simulink model "Frame"  (R2021b)
settings: Solver=FixedStepAuto  StartTime=0.0  StopTime=10  FixedStep=Ts  RelTol=1e-3
model workspace (MAT data in the model file):
  Ts = 0.005
values from neighbouring files (symbols this model uses):
  CODE = str2num(app.InsrerlecodebarresvirguleEditField.Value)    [cao.m]
undefined symbols (not defined in the file or in its folder): alpha_c, amp, AnimActive, couple, courbure, dx_c, dz_c, F_s, filtre, freq, I_0, J_s, photod, ref, theta_c, w_0
libraries: simulink x2
settings Model: Creator=GUBED49  LastModifiedBy=billy
settings DataIOCC: SaveFormat=Array  SignalLogging=off  DSMLogging=off  ReturnWorkspaceOutputs=off

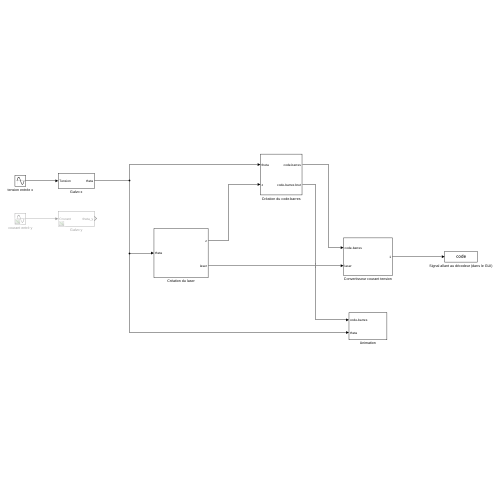
[thumbnail: Simulink's stored preview of the top-level diagram]
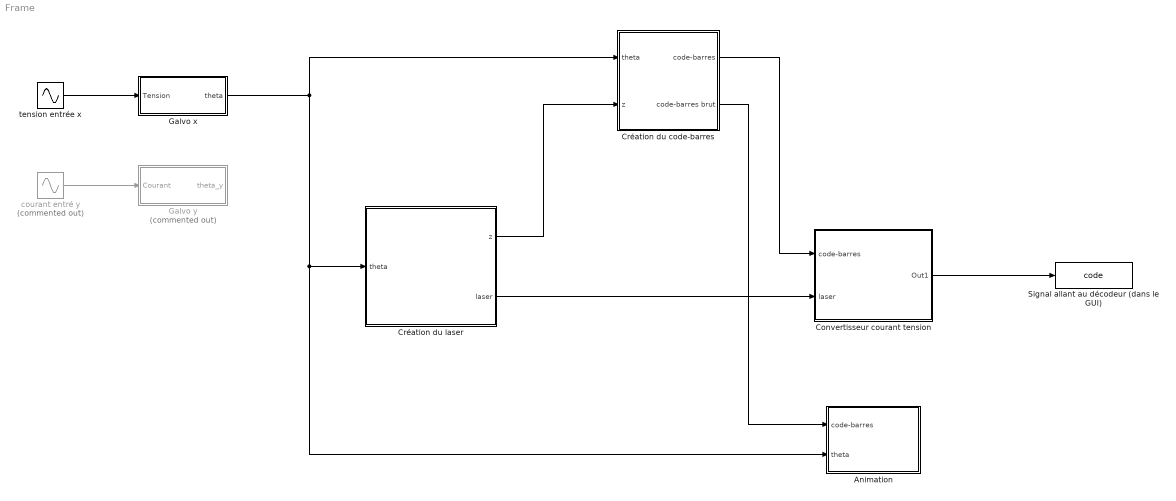
== system Frame ==
  Animation : Subsystem
  Convertisseur courant tension : Subsystem
  Création du code-barres : Subsystem
  Création du laser : Subsystem
  Galvo x : Subsystem
  Galvo y : Subsystem  Commented=on
  Signal allant au décodeur (dans le GUI) : ToWorkspace  VariableName=code  SampleTime=-1
  courant entré y : Sin  Commented=on  Amplitude=amp  Frequency=freq*2*pi  SampleTime=0
  tension entrée x : Sin  Amplitude=amp  Frequency=freq  SampleTime=0
  wires:
  tension entrée x/1 -> Galvo x/1(Tension)
  Galvo x/1(theta) -> Animation/2(theta), Création du laser/1(theta), Création du code-barres/1(theta)
  Création du laser/1(z) -> Création du code-barres/2(z)
  Création du code-barres/1(code-barres) -> Convertisseur courant tension/1(code-barres)
  Création du laser/2(laser) -> Convertisseur courant tension/2(laser)
  Convertisseur courant tension/1(Out1) -> Signal allant au décodeur (dans le GUI)/1
  courant entré y/1 -> Galvo y/1(Courant)
  Création du code-barres/2(code-barres brut) -> Animation/1(code-barres)

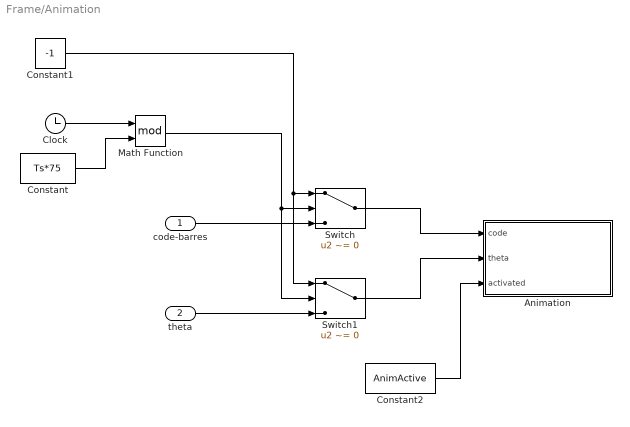
== system Frame/Animation ==
  code-barres : Inport
  theta : Inport  Port=2
  Animation : MATLAB Function  TreatAsAtomicUnit=on
  Clock : Clock
  Constant : Constant  Value=Ts*75
  Constant1 : Constant  Value=-1
  Constant2 : Constant  Value=AnimActive
  Math Function : Math  Operator=mod  SaturateOnIntegerOverflow=on
  Switch : Switch  Criteria=u2 ~= 0  Threshold=10
  Switch1 : Switch  Criteria=u2 ~= 0  Threshold=10
  wires:
  Switch1/1 -> Animation/2(theta)
  Math Function/1 -> Switch1/2, Switch/2
  Clock/1 -> Math Function/1
  Constant1/1 -> Switch1/1, Switch/1
  Constant/1 -> Math Function/2
  Switch/1 -> Animation/1(code)
  theta/1 -> Switch1/3
  code-barres/1 -> Switch/3
  Constant2/1 -> Animation/3(activated)

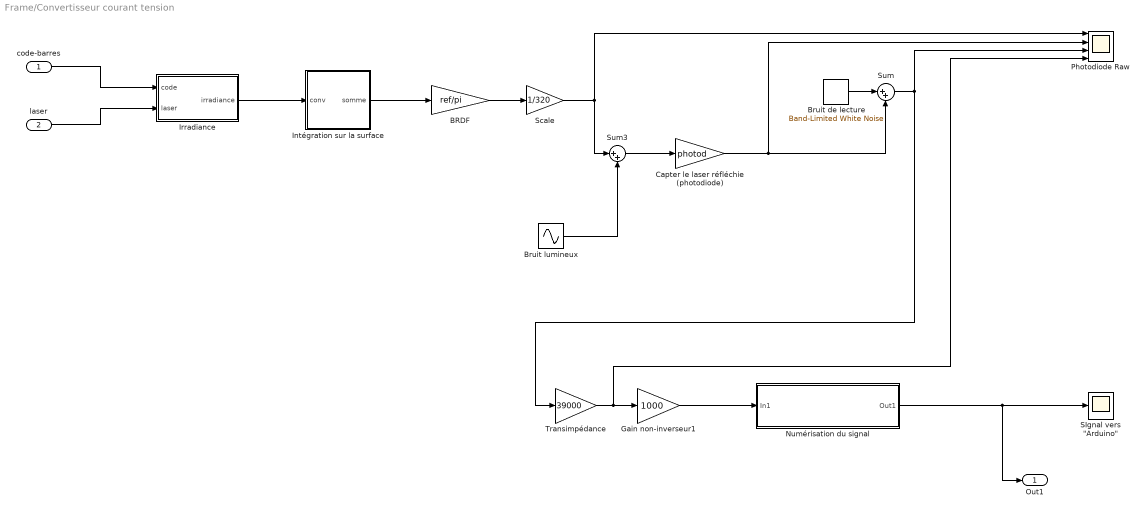
== system Frame/Convertisseur courant tension ==
  code-barres : Inport
  laser : Inport  Port=2
  BRDF : Gain  Gain=ref/pi
  Bruit de lecture : simulink/Sources/Band-Limited White Noise  Cov=[0.00000000000000001]  Ts=0.1  seed=[23341]
  Bruit lumineux : Sin  Amplitude=0.000001  Bias=0.000  Frequency=7  SampleTime=0
  Capter le laser réfléchie (photodiode) : Gain  Gain=photod
  Gain non-inverseur1 : Gain  Gain=1000
  Intégration sur la surface : MATLAB Function  TreatAsAtomicUnit=on
  Irradiance : MATLAB Function  TreatAsAtomicUnit=on
  Numérisation du signal : Subsystem
  Photodiode Raw : Scope  NumInputPorts=4
  "SIgnal vers \"Arduino\"" : Scope
  Scale : Gain  Gain=1/320
  Sum : Sum  Inputs=|++
  Sum3 : Sum  Inputs=|++
  Transimpédance : Gain  Gain=39000
  Out1 : Outport
  wires:
  Sum3/1 -> Capter le laser réfléchie (photodiode)/1
  Intégration sur la surface/1(somme) -> BRDF/1
  Bruit lumineux/1 -> Sum3/2
  Capter le laser réfléchie (photodiode)/1 -> Photodiode Raw/2, Sum/2
  Numérisation du signal/1(Out1) -> "SIgnal vers \"Arduino\""/1, Out1/1
  Gain non-inverseur1/1 -> Numérisation du signal/1(In1)
  BRDF/1 -> Scale/1
  Scale/1 -> Sum3/1, Photodiode Raw/1
  Bruit de lecture/1 -> Sum/1
  Sum/1 -> Transimpédance/1, Photodiode Raw/3
  laser/1 -> Irradiance/2(laser)
  code-barres/1 -> Irradiance/1(code)
  Irradiance/1(irradiance) -> Intégration sur la surface/1(conv)
  Transimpédance/1 -> Gain non-inverseur1/1, Photodiode Raw/4

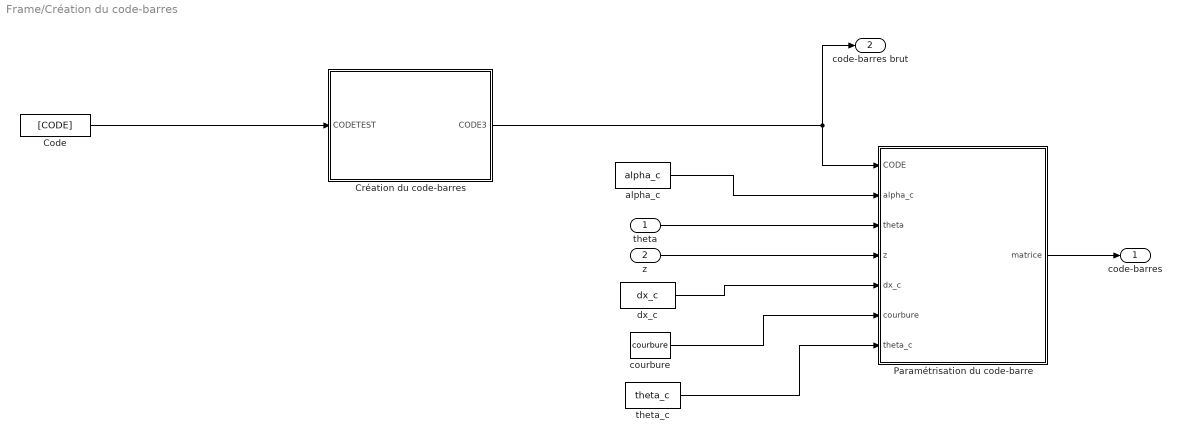
== system Frame/Création du code-barres ==
  theta : Inport
  z : Inport  Port=2
  Code : Constant  Value=[CODE]
  Création du code-barres : MATLAB Function  TreatAsAtomicUnit=on
  Paramétrisation du code-barre : MATLAB Function  TreatAsAtomicUnit=on
  alpha_c : Constant  Value=alpha_c
  courbure : Constant  Value=courbure
  dx_c : Constant  Value=dx_c
  theta_c : Constant  Value=theta_c
  code-barres : Outport
  code-barres brut : Outport  Port=2
  wires:
  Création du code-barres/1(CODE3) -> code-barres brut/1, Paramétrisation du code-barre/1(CODE)
  alpha_c/1 -> Paramétrisation du code-barre/2(alpha_c)
  dx_c/1 -> Paramétrisation du code-barre/5(dx_c)
  theta/1 -> Paramétrisation du code-barre/3(theta)
  z/1 -> Paramétrisation du code-barre/4(z)
  Paramétrisation du code-barre/1(matrice) -> code-barres/1
  courbure/1 -> Paramétrisation du code-barre/6(courbure)
  Code/1 -> Création du code-barres/1(CODETEST)
  theta_c/1 -> Paramétrisation du code-barre/7(theta_c)

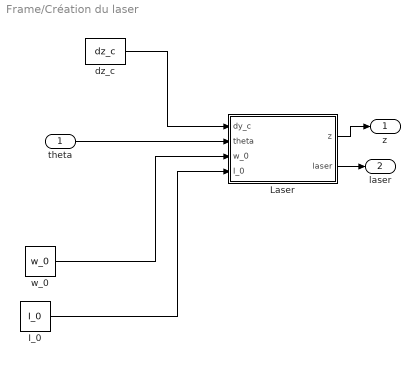
== system Frame/Création du laser ==
  theta : Inport
  I_0 : Constant  Value=I_0
  Laser : MATLAB Function  TreatAsAtomicUnit=on
  dz_c : Constant  Value=dz_c
  w_0 : Constant  Value=w_0
  z : Outport
  laser : Outport  Port=2
  wires:
  theta/1 -> Laser/2(theta)
  w_0/1 -> Laser/3(w_0)
  I_0/1 -> Laser/4(I_0)
  dz_c/1 -> Laser/1(dy_c)
  Laser/2(laser) -> laser/1
  Laser/1(z) -> z/1

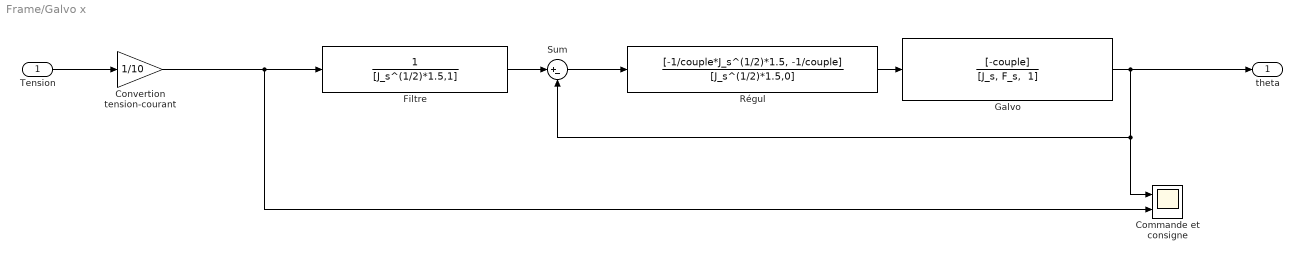
== system Frame/Galvo x ==
  Tension : Inport
  Commande et consigne : Scope  NumInputPorts=2
  Convertion tension-courant : Gain  Gain=1/10
  Filtre : TransferFcn  Numerator=1  Denominator=[J_s^(1/2)*1.5,1]
  "Galvo " : TransferFcn  Numerator=[-couple]  Denominator="[J_s, F_s,  1]"
  Régul : TransferFcn  Numerator=[-1/couple*J_s^(1/2)*1.5, -1/couple]  Denominator=[J_s^(1/2)*1.5,0]
  Sum : Sum  Inputs=|+-
  theta : Outport
  wires:
  Tension/1 -> Convertion tension-courant/1
  Sum/1 -> Régul/1
  "Galvo "/1 -> Commande et consigne/1, Sum/2, theta/1
  Régul/1 -> "Galvo "/1
  Convertion tension-courant/1 -> Commande et consigne/2, Filtre/1
  Filtre/1 -> Sum/1

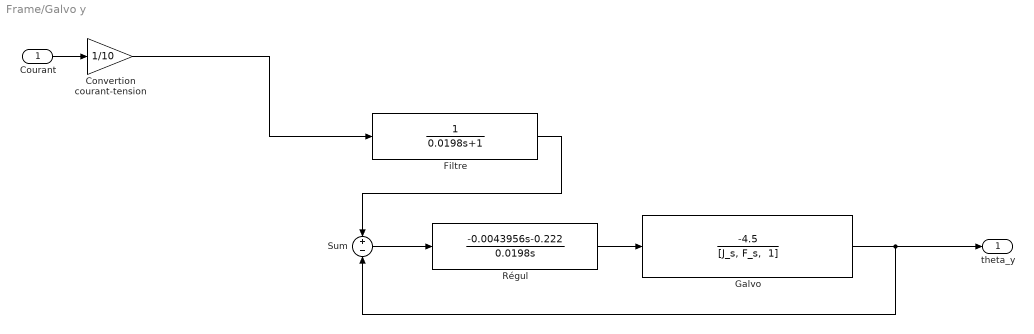
== system Frame/Galvo y ==
  Courant : Inport
  Convertion courant-tension : Gain  Gain=1/10
  Filtre : TransferFcn  Numerator=1  Denominator=[0.0198,1]
  "Galvo " : TransferFcn  Numerator=[-4.5]  Denominator="[J_s, F_s,  1]"
  Régul : TransferFcn  Numerator=[-0.0043956, -0.222]  Denominator=[0.0198,0]
  Sum : Sum  Inputs=+|-
  theta_y : Outport
  wires:
  Courant/1 -> Convertion courant-tension/1
  Sum/1 -> Régul/1
  "Galvo "/1 -> Sum/2, theta_y/1
  Régul/1 -> "Galvo "/1
  Convertion courant-tension/1 -> Filtre/1
  Filtre/1 -> Sum/1

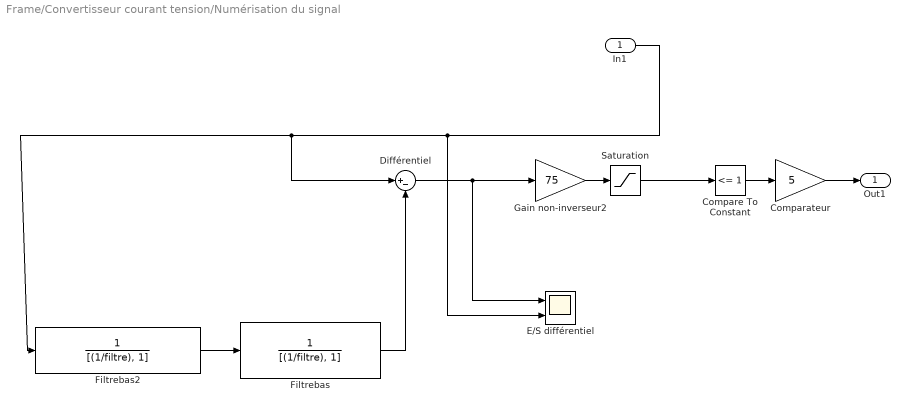
== system Frame/Convertisseur courant tension/Numérisation du signal ==
  In1 : Inport
  Comparateur : Gain  Gain=5
  Compare To Constant : simulink/Logic and Bit Operations/Compare To Constant  relop=<=  const=1  OutDataTypeStr=boolean
  Différentiel : Sum  Inputs=|+-
  E/S différentiel : Scope  NumInputPorts=2
  Filtrebas : TransferFcn  Numerator=1  Denominator=[(1/filtre), 1]
  Filtrebas2 : TransferFcn  Numerator=1  Denominator=[(1/filtre), 1]
  Gain non-inverseur2 : Gain  Gain=75
  Saturation : Saturate  UpperLimit=5  LowerLimit=0
  Out1 : Outport
  wires:
  Gain non-inverseur2/1 -> Saturation/1
  Filtrebas2/1 -> Filtrebas/1
  In1/1 -> E/S différentiel/2, Filtrebas2/1, Différentiel/1
  Compare To Constant/1 -> Comparateur/1
  Différentiel/1 -> E/S différentiel/1, Gain non-inverseur2/1
  Saturation/1 -> Compare To Constant/1
  Filtrebas/1 -> Différentiel/2
  Comparateur/1 -> Out1/1

== matlab function Frame/Création du laser/Laser ==
  data: z output; dy_c input; laser output size=[100 100]; theta input; w_0 input; I_0 input
function [z, laser] = fcn(dy_c, theta, w_0, I_0)
GRAND=10;
z=dy_c/cosd(theta+0.000000000001);
z_0 = (pi*(w_0^(-2))^2)/(650*10^(-9));
w = (w_0*sqrt(1+(z/z_0)^2));
pas=0.033/GRAND;

laser4=zeros(5*GRAND, 5*GRAND);
for col= 1 : 5*GRAND
    for row = 1 : 5*GRAND
        col_1= (col*pas)-pas;
        row_1= (row*pas)-pas;
        rayon=sqrt(row_1^2+col_1^2);
laser4(row, col) = (I_0*(w_0/w)^(2)*exp((-2*((rayon)^2))/(w^2)));

    end
end
laser3=fliplr(laser4);
laser1=flipud(laser4);
laser2=fliplr(laser1);
laser=[laser2 laser1; laser3 laser4];

== matlab function Frame/Création du code-barres/Création du code-barres ==
  data: CODETEST input; CODE3 output
function CODE3 = fcn(CODETEST)
GRAND=10;

GAUCHE = [0 0 0 1 1 0 1; 0 0 1 1 0 0 1; 0 0 1 0 0 1 1; 0 1 1 1 1 0 1; 0 1 0 0 0 1 1; 0 1 1 0 0 0 1; 0 1 0 1 1 1 1; 0 1 1 1 0 1 1; 0 1 1 0 1 1 1; 0 0 0 1 0 1 1];
DROITE = [1 1 1 0 0 1 0; 1 1 0 0 1 1 0; 1 1 0 1 1 0 0; 1 0 0 0 0 1 0; 1 0 1 1 1 0 0; 1 0 0 1 1 1 0; 1 0 1 0 0 0 0; 1 0 0 0 1 0 0; 1 0 0 1 0 0 0; 1 1 1 0 1 0 0];



%Génération du code-barres

START=[ 1 0 1];
END=[1 0 1];
MIDDLE=[0 1 0 1 0];
QUIET=zeros(1,9);
CGAUCHE=[];
CDROITE=[];



for i = 1: 6
    val=CODETEST(i);
    val=val+1;
    CGAUCHE = [CGAUCHE,GAUCHE(val,:)];
end

for j = 7 : 12
    val=CODETEST(j);
    val=val+1;
    CDROITE = [CDROITE, DROITE(val, :)];
end 

CGAUCHE=transpose(CGAUCHE);
CDROITE=transpose(CDROITE);
CGAUCHE=reshape(CGAUCHE,1,42);
CDROITE=reshape(CDROITE,1,42);
CODE=[ QUIET START CGAUCHE MIDDLE CDROITE END QUIET];
CODEBAS= [ QUIET START zeros([1 42]) MIDDLE zeros([1 42]) END QUIET];




CODE=(repelem(CODE,GRAND));
CODEBAS=(repelem(CODEBAS,GRAND));

for i=1:(77*GRAND)
    CODE2=[CODE;CODE(1,:)];
end
for i=1:(5*GRAND)
    CODE3=[CODE2;CODEBAS(1,:)];
end

== matlab function Frame/Animation/Animation ==
  settings: updateMethod=DISCRETE  sampleTime=Ts
  data: code input; theta input; activated input
function fcn(code,theta,activated)
persistent f
coder.extrinsic('imshow')

if ~activated
    return
end

if isempty(f)
    f = figure('Name', 'Animation de la simulation', 'IntegerHandle','off');
end

if code == -1
    return
end

if ~ishandle(f)
    return
end

set(0, 'CurrentFigure', f)

code = repelem(code(1:2,:), 200,1);

% Generate laser dot
imsize = flip(size(code));
[columnsInImage, rowsInImage] = meshgrid(1:imsize(1), 1:imsize(2));
centerY = floor(imsize(2)/2);
centerX = (imsize(1)/2) * (sind(theta)/0.23 + 1); % Trop fatigué pour comprendre pourquoi ca marche mais ca marche
radius = 10;
circlePixels = (rowsInImage - centerY).^2 ...
     + (columnsInImage - centerX).^2 <= radius.^2;

% Merge images and show
im = (circlePixels*2+code)./2;
imshow(im, Colormap=[1 1 1; 0 0 0; 1 0 0]);

== matlab function Frame/Création du code-barres/Paramétrisation du code-barre ==
  data: CODE input; matrice output; alpha_c input; theta input; z input; dx_c input; courbure input; theta_c input
function matrice    = fcn(CODE, alpha_c, theta,z, dx_c, courbure,theta_c)
GRAND=10;

dim_theta = cosd(theta_c); %diminution de la largeur d'une bande dans le référentiel du laser par l'angle theta_c

x = (sind(theta+0.00000000001)*z); %x' dans le séminaire
x_c = x/cosd(alpha_c);

pas=0.033/GRAND; %Largeur voulue d'une colonne

dim_R = cos(x_c/courbure); %diminution de la largeur d'une bande dans le référentiel du laser par la courbure plus on s'éloigne du centre


decal= round(dim_R*dim_theta*(dx_c/cosd(alpha_c))/pas);

c1 = round(dim_R*dim_theta*(x/cosd(alpha_c))/pas);

c = c1+decal;
if c < -56*GRAND
c=-56*GRAND;
end
if c > 56*GRAND
    c=56*GRAND;
end

matrice=CODE(:, (57*GRAND)+c);

== matlab function Frame/Convertisseur courant tension/Intégration sur la surface ==
  data: conv input; somme output
function somme = fcn(conv)
somme=(mean(mean(conv(:))))/20;

== matlab function Frame/Convertisseur courant tension/Irradiance ==
  data: code input; laser input; irradiance output
function irradiance = fcn(code,laser)
irradiance = conv2(code, laser);
